simulink library "milstd_library"  (Simulink 6.0)
settings: Solver=ode45  SolverMode=SingleTasking  StartTime=0.0  StopTime=10.0  RelTol=1e-3
undefined symbols (not defined in the file or in its folder): milstd
libraries: simulink x13, commutil2 x11, dspsigattribs x6, dspbuff3 x5, commcnvcod2 x4, commseqgen2 x3, milstd_library x3, dspsigops x3, dspsrcs4 x3, dspmtrx3 x2, commdigbbndpm2 x2, commblkintrlv2 x2
settings Model: Creator=arodrigu  LastModifiedBy=arodrigu
settings DataIOCC: SignalLoggingName=logsOut
settings OptimizationCC: BooleanDataType=off
settings DebuggingCC: CheckExecutionContextPreStartOutputMsg=on  CheckExecutionContextRuntimeOutputMsg=on  SolverPrmCheckMsg=none
settings HardwareCC: TargetUnknown=on
settings ModelReferenceCC: UpdateModelReferenceTargets=IfOutOfDate
settings SFSimCC: SFSimApplyToAllLibs=on  SFSimBuildMode=Incremental

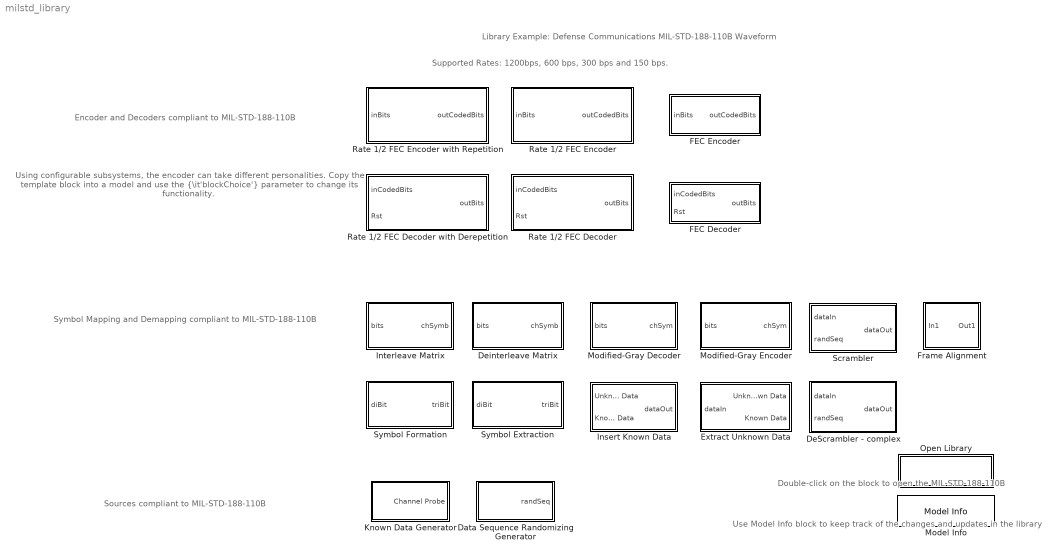
== system milstd_library ==
  note: Library Example: Defense Communications MIL-STD-188-110B Waveform
  note: Encoder and Decoders
      | compliant to
      | MIL-STD-188-110B
  note: Symbol Mapping and Demapping
      | compliant to
      | MIL-STD-188-110B
  note: Sources
      | compliant to
      | MIL-STD-188-110B
  note: Using configurable subsystems,
      | the encoder can take different
      | personalities. Copy the template block
      | into a model and use the {\it'blockChoice'}
      | parameter to change its functionality.
  note: Supported Rates: 1200bps, 600 bps, 300 bps and 150 bps.
  note: Use Model Info block to keep track of
      | the changes and updates in the library
  note: Double-click on the block
      | to open the MIL-STD-188-110B
  Data Sequence Randomizing Generator : Subsystem  PropExecContextAcrossSSBoundary=on
  DeScrambler - complex : Subsystem  PropExecContextAcrossSSBoundary=on
      mask Display:
      | disp('Descrambler\n')
      | port_label('input',1,'');
      | port_label('input',2,'rndSeq');
  Deinterleave Matrix : Subsystem  PropExecContextAcrossSSBoundary=on
      mask Display: disp('Deinterleave\nMatrix')
  Extract Unknown Data : Subsystem  PropExecContextAcrossSSBoundary=on
      mask Display: disp('Extract\nUnknown Data')
  FEC Decoder : Subsystem  BlockChoice=Rate 1/2 FEC Decoder  PropExecContextAcrossSSBoundary=on
      settings: TemplateBlock=self  MemberBlocks=Rate 1/2 FEC Decoder,Rate 1/2 FEC Decoder with Derepetition
  FEC Encoder : Subsystem  BlockChoice=Rate 1/2 FEC Encoder  PropExecContextAcrossSSBoundary=on
      settings: TemplateBlock=self  MemberBlocks=Rate 1/2 FEC Encoder,Rate 1/2 FEC Encoder with Repetition
  Frame Alignment : Subsystem  PropExecContextAcrossSSBoundary=on
      mask Display: disp('Frame\nAlignment')
  Insert Known Data : Subsystem  PropExecContextAcrossSSBoundary=on
      mask Display: disp('Insert\nKnown Data')
  Interleave Matrix : Subsystem  PropExecContextAcrossSSBoundary=on
      mask Display: disp('Interleave\nMatrix')
  Known Data Generator : Subsystem  PropExecContextAcrossSSBoundary=on
  Model Info : simulink/Model-Wide Utilities/Model Info  InitialBlockCM=None  BlockCM=None  Frame=on  DisplayStringWithTags=|  HorizontalTextAlignment=Center  LeftAlignmentValue=0.5  SourceBlockDiagram=milstd_library  TagMaxNumber=20
      | Model Info
      | Model version: %<ModelVersion>
  Modified-Gray Decoder : Subsystem  PropExecContextAcrossSSBoundary=on
      mask Display: disp('Bits to\nChannel\nSymbols')
  Modified-Gray Encoder : Subsystem  PropExecContextAcrossSSBoundary=on
      mask Type: Modified-Gray Encoder
      mask Display: disp('Channel\nSymbols\nto Bits')
  Open Library : Subsystem  PropExecContextAcrossSSBoundary=on
      settings: OpenFcn=open('milstd_188110bmodel.mdl');
      mask Display: disp('MIL-STD-188-110B\nModel')
  Rate 1/2 FEC Decoder : Subsystem  PropExecContextAcrossSSBoundary=on
      mask Display: disp('Rate 1/2\nFEC Decoding:\nViterbi Decoder');
  Rate 1/2 FEC Decoder with Derepetition : Subsystem  PropExecContextAcrossSSBoundary=on
      mask Display: disp('Rate 1/2\nFEC Decoding:\nViterbi Decoder\nwith Derepetition');
  Rate 1/2 FEC Encoder : Subsystem  PropExecContextAcrossSSBoundary=on
      mask Display: disp('Rate 1/2 FEC\nEncoder')
  Rate 1/2 FEC Encoder with Repetition : Subsystem  PropExecContextAcrossSSBoundary=on
      mask Display: disp('Rate 1/2 FEC\nEncoder\n with Repetition')
  Scrambler : Subsystem  PropExecContextAcrossSSBoundary=on
      mask Display:
      | disp('Scrambler')
      | port_label('input',1,'');
      | port_label('input',2,'rndSeq');
  Symbol Extraction : Subsystem  PropExecContextAcrossSSBoundary=on
      mask Display: disp('Symbol\nExtraction:\nUnknown Data')
  Symbol Formation : Subsystem  PropExecContextAcrossSSBoundary=on
      mask Display: disp('Symbol\nFormation:\nUnknown Data')

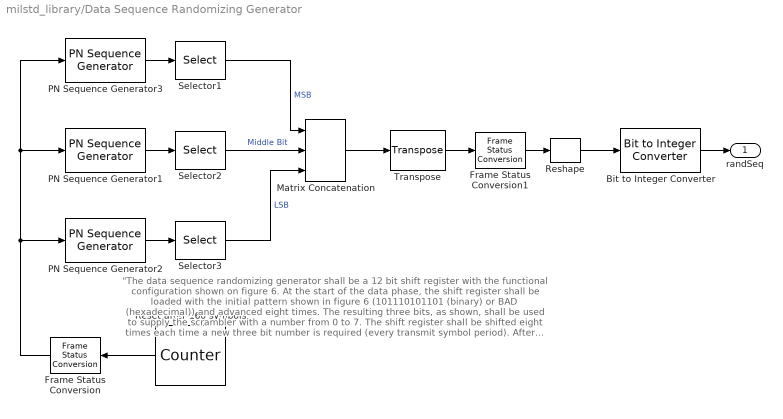
== system milstd_library/Data Sequence Randomizing Generator ==
  note: "The  data  sequence  randomizing  generator  shall  be  a  12  bit  shift  register  with  the  functional
      | configuration shown on figure 6. At the start of the data phase, the shift register shall be loaded
      | with the initial pattern shown in figure 6 (101110101101 (binary) or BAD (hexadecimal)) and
      | advanced eight times. The resulting three bits, as shown, shall be used to supply the scrambler
      | with a number from 0 to 7. The shift register shall be shifted eight times each time a new three
      | bit number is required  (every transmit symbol period). After 160 transmit symbols, the shift
      | register shall be reset to BAD (hexadecimal) prior to the eight shifts. "
      |
      | Source: MIL-STD-188-110B: Interoperability and Performance Standards for Data Modems,
      | U.S. Department of Defense, 2000.
  Bit to Integer Converter : commutil2/Bit to Integer Converter  nbits=3
  Frame Status Conversion : dspsigattribs/Frame Status Conversion  Orientation=left  growRefPort=off  outframe=Frame-based
  Frame Status Conversion1 : dspsigattribs/Frame Status Conversion  growRefPort=off  outframe=Frame-based
  Matrix Concatenation : simulink/Math Operations/Matrix Concatenation  numInports=3  catMethod=Horizontal
  PN Sequence Generator1 : commseqgen2/PN Sequence Generator  poly=[12 6 4 1 0]  ini_sta=[zeros(1,11) 1]  shift=3664  Ts=1/2400/8  frameBased=on  sampPerFrame=40*8  reset=on
  PN Sequence Generator2 : commseqgen2/PN Sequence Generator  poly=[12 6 4 1 0]  ini_sta=[zeros(1,11) 1]  shift=1506  Ts=1/2400/8  frameBased=on  sampPerFrame=40*8  reset=on
  PN Sequence Generator3 : commseqgen2/PN Sequence Generator  poly=[12 6 4 1 0]  ini_sta=[zeros(1,11) 1]  shift=3663  Ts=1/2400/8  frameBased=on  sampPerFrame=40*8  reset=on
  Reset after 160 symbols : dspswit3/Counter  Orientation=left  Direction=Down  CountEvent=Free running  CounterSize=User defined  MaxCount=160/40+1  InitialCount=160/40+1  Output=Hit  HitValue=1  ResetInput=off  SamplesPerFrame=1  Ts=40/2400  CntDtype=double  HitDtype=Logical
  Reshape : simulink/Math Operations/Reshape  OutputDimensionality=Column vector  OutputDimensions=[1,1]
  Selector1 : Selector  Elements=[8:8:40*8]  InputPortWidth=40*8
  Selector2 : Selector  Elements=[8:8:40*8]  InputPortWidth=40*8
  Selector3 : Selector  Elements=[8:8:40*8]  InputPortWidth=40*8
  Transpose : dspmtrx3/Transpose  Hermitian=off  overflowFlag=on
  randSeq : Outport
  wires:
  PN Sequence Generator2/1 -> Selector3/1
  PN Sequence Generator1/1 -> Selector2/1
  PN Sequence Generator3/1 -> Selector1/1
  Selector1/1 -> Matrix Concatenation/1  "MSB"
  Selector2/1 -> Matrix Concatenation/2  "Middle Bit"
  Selector3/1 -> Matrix Concatenation/3  "LSB"
  Bit to Integer Converter/1 -> randSeq/1
  Reset after 160 symbols/1 -> Frame Status Conversion/1
  Frame Status Conversion/1 -> PN Sequence Generator3/1, PN Sequence Generator1/1, PN Sequence Generator2/1
  Matrix Concatenation/1 -> Transpose/1
  Transpose/1 -> Frame Status Conversion1/1
  Reshape/1 -> Bit to Integer Converter/1
  Frame Status Conversion1/1 -> Reshape/1

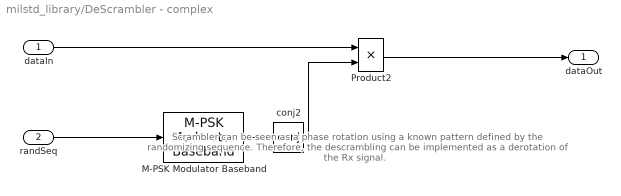
== system milstd_library/DeScrambler - complex ==
  note: Scrambler can be seen as a phase rotation using a known
      | pattern defined by the randomizing sequence. Therefore,
      | the descrambling can be implemented as a derotation of the
      | Rx signal.
  dataIn : Inport  LatchInput=off
  randSeq : Inport  Port=2  LatchInput=off
  M-PSK Modulator Baseband : commdigbbndpm2/M-PSK Modulator Baseband  M=8  InType=Integer  Enc=Binary  Ph=0  numSamp=1
  Product2 : Product  SaturateOnIntegerOverflow=on  InputSameDT=on
  conj2 : Math  Operator=conj  SaturateOnIntegerOverflow=on
  dataOut : Outport
  wires:
  Product2/1 -> dataOut/1
  conj2/1 -> Product2/2
  M-PSK Modulator Baseband/1 -> conj2/1
  randSeq/1 -> M-PSK Modulator Baseband/1
  dataIn/1 -> Product2/1

== system milstd_library/Deinterleave Matrix ==
  bits : Inport  LatchInput=off
  Buffer : dspbuff3/Buffer  N=milstd.rate*milstd.repFactor*2*0.2  V=0  ic=0
  General Block Deinterleaver : commblkintrlv2/General Block Deinterleaver  elements=milstd.interTable %Column vector
  chSymb : Outport
  wires:
  bits/1 -> General Block Deinterleaver/1
  General Block Deinterleaver/1 -> Buffer/1
  Buffer/1 -> chSymb/1

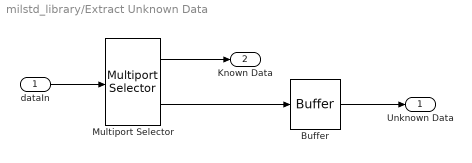
== system milstd_library/Extract Unknown Data ==
  dataIn : Inport  LatchInput=off
  Buffer : dspbuff3/Buffer  N=milstd.rate*2*milstd.interl*milstd.repFactor*3/milstd.bitsToSym  V=0  ic=0
  Multiport Selector : dspindex/Multiport Selector  rowsOrCols=Rows  idxCellArray={ [1:60],[61:120]}  idxErrMode=Clip Index
  Unknown Data : Outport
  Known Data : Outport  Port=2
  wires:
  dataIn/1 -> Multiport Selector/1
  Multiport Selector/1 -> Known Data/1
  Multiport Selector/2 -> Buffer/1
  Buffer/1 -> Unknown Data/1

== system milstd_library/FEC Decoder ==
  inCodedBits : Inport  LatchInput=off
  Rst : Inport  Port=2  LatchInput=off
  Rate 1/2 FEC Decoder : milstd_library/Rate 1//2 FEC Decoder
  outBits : Outport
  wires:
  inCodedBits/1 -> Rate 1/2 FEC Decoder/1
  Rst/1 -> Rate 1/2 FEC Decoder/2
  Rate 1/2 FEC Decoder/1 -> outBits/1

== system milstd_library/FEC Encoder ==
  inBits : Inport  LatchInput=off
  Rate 1/2 FEC Encoder : milstd_library/Rate 1//2 FEC Encoder
  outCodedBits : Outport
  wires:
  inBits/1 -> Rate 1/2 FEC Encoder/1
  Rate 1/2 FEC Encoder/1 -> outCodedBits/1

== system milstd_library/Frame Alignment ==
  note: This block collects a block
      | of data equal to size of the interleaver
      | matrix depending on the data rate and
      | interleaver length
  note: This extra delay is intended to
      | align the signal to the beginning of
      | the interleaver frame
  In1 : Inport  LatchInput=off
  Buffer : dspbuff3/Buffer  N=1200*milstd.interl  V=0  ic=0
  Delay : dspsigops/Delay  dly_unit=Samples  delay=1200*milstd.interl-20  ic_detail=off  dif_ic_for_ch=off  dif_ic_for_dly=off  ic=0  reset_popup=None
  Out1 : Outport
  wires:
  Delay/1 -> Buffer/1
  Buffer/1 -> Out1/1
  In1/1 -> Delay/1

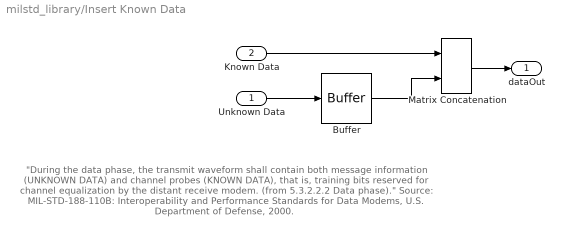
== system milstd_library/Insert Known Data ==
  note: "During  the  data  phase,  the  transmit  waveform  shall  contain  both  message  information
      | (UNKNOWN DATA) and channel probes (KNOWN DATA), that is, training bits reserved for
      | channel equalization by the distant receive modem. (from 5.3.2.2.2 Data phase)."
      |
      | Source: MIL-STD-188-110B: Interoperability and Performance Standards for Data Modems,
      | U.S. Department of Defense, 2000.
  Unknown Data : Inport  LatchInput=off
  Known Data : Inport  Port=2  LatchInput=off
  Buffer : dspbuff3/Buffer  N=20*3  V=0  ic=0
  Matrix Concatenation : simulink/Math Operations/Matrix Concatenation  numInports=2  catMethod=Vertical
  dataOut : Outport
  wires:
  Buffer/1 -> Matrix Concatenation/2
  Known Data/1 -> Matrix Concatenation/1
  Matrix Concatenation/1 -> dataOut/1
  Unknown Data/1 -> Buffer/1

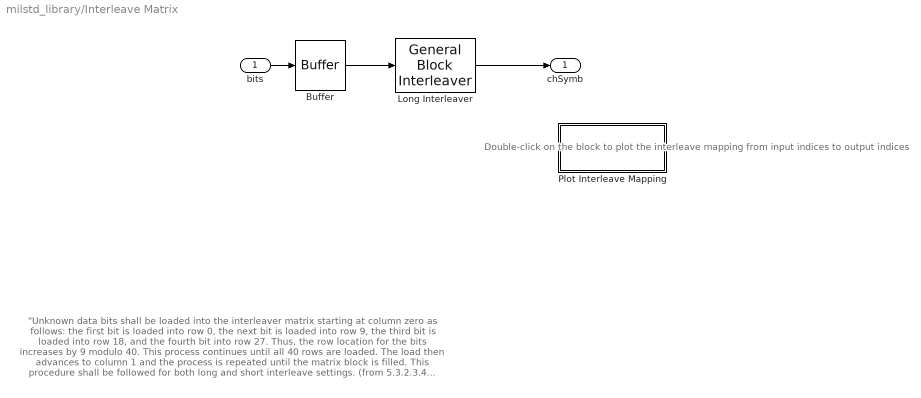
== system milstd_library/Interleave Matrix ==
  note: "Unknown data bits shall be loaded into the interleaver matrix starting at column zero as follows:
      | the first bit is loaded into row 0, the next bit is loaded into row 9, the third bit is loaded into row 18, and the fourth
      | bit into row 27. Thus, the row location for the bits increases by 9 modulo 40. This process continues until all 40 rows
      | are loaded. The load then advances to column 1 and the process is repeated until the matrix block is filled. This procedure
      | shall be followed for both long and short interleave settings. (from 5.3.2.3.4 Interleave load).
      |
      | To maintain the interleave delay at a constant value, the block size shall be scaled by bit rate. TABLES X lists the interleaver
      | matrix dimensions (rows and columns) that shall be allocated for each requir d bit rate and interleave delay.
      |
      | The fetching sequence for all rates shall start with the first bit being taken from row zero, column zero. The location of
      | each successive fetched bit shall be determined by incrementing the row by one and decrementing the column
      | number by 17 (modulo number of columns in the interleaver matrix).  (from 5.3.2.3.5 Interleave fetch)."
      |
      | Source: MIL-STD-188-110B: Interoperability and Performance Standards for Data Modems, U.S. Department of Defense, 2000.
  note: Double-click on the block to
      | plot the interleave mapping from
      | input indices to output indices
  bits : Inport  LatchInput=off
  Buffer : dspbuff3/Buffer  N=milstd.rate*milstd.interl*milstd.repFactor*2 % x2 because of coding rate  V=0  ic=0
  Long Interleaver : commblkintrlv2/General Block Interleaver  elements=milstd.interTable %Column vector
  Plot Interleave Mapping : Subsystem  PropExecContextAcrossSSBoundary=on
      settings: OpenFcn=|
      | figure;
      | numRow = 40;
      | numCol = length(milstd.interTable)/numRow;
      | plot([0:numRow*numCol-1],milstd.interTable,'b.');
      | axis([0 numRow*numCol-1 0 numRow*numCol-1]);
      | title('Interleaver Mapping');
      | xlabel('Input index');
      | ylabel('Output index');
      mask Display: disp('Interleave\nMapping')
  chSymb : Outport
  wires:
  Long Interleaver/1 -> chSymb/1
  Buffer/1 -> Long Interleaver/1
  bits/1 -> Buffer/1

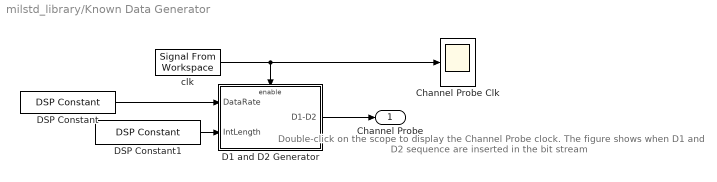
== system milstd_library/Known Data Generator ==
  note: Double-click on the scope to display
      | the Channel Probe clock. The figure shows
      | when D1 and D2 sequence are inserted in
      | the bit stream
  Channel Probe Clk : Scope
      settings: TimeRange=19.2  DataFormat=Structure
  D1 and D2 Generator : Subsystem  PropExecContextAcrossSSBoundary=on
      mask init:
      | % Loads lookup table for D1 and D2 bits in preamble sequence
      | % according to MIL-STD-188-110B TABLE XV
      | % D1 Lookup table:
      | D1Table = ones(7,2);
      | D1Table(:,1) = [ 7 6 6 6 6 7 7]';
      | D1Table(:,2) = [ 0 4 4 4 4 5 5]';
      | 
      | % D1 Lookup table:
      | D2Table = ones(7,2);
      | D2Table(:,1) = [6 4 5 6 7 4 5]';
      | D2Table(:,2) = [0 4 5 6 7 4 5]';
  DSP Constant : dspsrcs4/DSP Constant  Value=milstd.idxRate  SampleMode=Discrete  discreteOutput=Frame-based  continuousOutput=Sample-based  sampTime=1  framePeriod=20/1200  dataType=Inherit from 'Constant value'  wordLen=16  udDataType=sfix(16)  fracBitsMode=Best precision  numFracBits=15  InterpretAs1D=-inf  Ts=-inf  FramebasedOutput=-inf
  DSP Constant1 : dspsrcs4/DSP Constant  Value=milstd.idxInterl  SampleMode=Discrete  discreteOutput=Frame-based  continuousOutput=Sample-based  sampTime=1  framePeriod=20/1200  dataType=Inherit from 'Constant value'  wordLen=16  udDataType=sfix(16)  fracBitsMode=Best precision  numFracBits=15  InterpretAs1D=-inf  Ts=-inf  FramebasedOutput=-inf
  clk : dspsrcs4/Signal From Workspace  X="[1 1 zeros(1,1200*milstd.rate/20-2)]  %Channel rate is equal to 1200"  Ts=20/1200  nsamps=1  OutputAfterFinalValue=Cyclic repetition
  Channel Probe : Outport
  wires:
  clk/1 -> D1 and D2 Generator/Enable, Channel Probe Clk/1
  DSP Constant/1 -> D1 and D2 Generator/1(DataRate)
  DSP Constant1/1 -> D1 and D2 Generator/2(IntLength)
  D1 and D2 Generator/1(D1-D2) -> Channel Probe/1

== system milstd_library/Modified-Gray Decoder ==
  note: The bits obtained from the interleaver matrix shall be
      | grouped together as one, two, or three bit
      | entities that will be referred to as channel symbols.
  note: "Modified-Gray decoding of the 2400 bps, 4800 bps (tribit), and 75 bps (fixed frequency) 1200
      | bps (dibit) channel symbols shall be in accordance with tables XII and XIII respectively. "
      |
      | Source: MIL-STD-188-110B: Interoperability and Performance Standards for Data Modems, U.S. Department of Defense, 2000.
  bits : Inport  LatchInput=off
  Bits to Channel symbols : commutil2/Bit to Integer Converter  nbits=milstd.bitsToSym
  Data Mapper : commutil2/Data Mapper  MapMode=Binary to Gray  M=2^milstd.bitsToSym  MapVec=[0 1 3 2]
  Integer to Bit Converter : commutil2/Integer to Bit Converter  nbits=milstd.bitsToSym
  chSym : Outport
  wires:
  Data Mapper/1 -> Integer to Bit Converter/1
  bits/1 -> Bits to Channel symbols/1
  Integer to Bit Converter/1 -> chSym/1
  Bits to Channel symbols/1 -> Data Mapper/1

== system milstd_library/Modified-Gray Encoder ==
  bits : Inport  LatchInput=off
  Bits to Channel symbols : commutil2/Bit to Integer Converter  nbits=milstd.bitsToSym
  Data Mapper : commutil2/Data Mapper  MapMode=Gray to Binary  M=2^milstd.bitsToSym  MapVec=[0 1 3 2]
  Integer to Bit Converter : commutil2/Integer to Bit Converter  nbits=milstd.bitsToSym
  chSym : Outport
  wires:
  Bits to Channel symbols/1 -> Data Mapper/1
  Integer to Bit Converter/1 -> chSym/1
  bits/1 -> Bits to Channel symbols/1
  Data Mapper/1 -> Integer to Bit Converter/1

== system milstd_library/Open Library ==
  note: This subsystem is intentionally left empty

== system milstd_library/Rate 1/2 FEC Decoder ==
  inCodedBits : Inport  Orientation=left  LatchInput=off
  Rst : Inport  Orientation=left  Port=2  LatchInput=off
  Rate 1/2 Viterbi Decoder : commcnvcod2/Viterbi Decoder  Orientation=left  trellis=poly2trellis(7, [133 171])  dectype=Hard Decision  nsdecb=4  tbdepth=34  opmode=Continuous  reset=on
  outBits : Outport  Orientation=left
  wires:
  inCodedBits/1 -> Rate 1/2 Viterbi Decoder/1
  Rst/1 -> Rate 1/2 Viterbi Decoder/2
  Rate 1/2 Viterbi Decoder/1 -> outBits/1

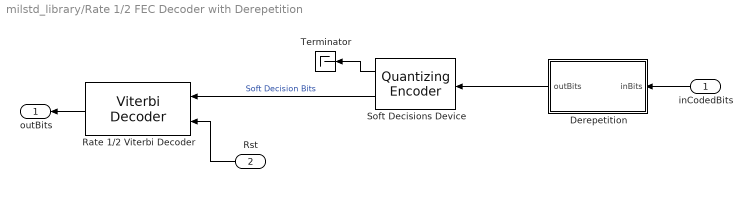
== system milstd_library/Rate 1/2 FEC Decoder with Derepetition ==
  inCodedBits : Inport  Orientation=left  LatchInput=off
  Rst : Inport  Orientation=left  Port=2  LatchInput=off
  Derepetition : Subsystem  Orientation=left  PropExecContextAcrossSSBoundary=on
      mask Display: disp('Derepetition')
  Rate 1/2 Viterbi Decoder : commcnvcod2/Viterbi Decoder  Orientation=left  trellis=poly2trellis(7, [133 171])  dectype=Soft Decision  nsdecb=2  tbdepth=34  opmode=Continuous  reset=on
  Soft Decisions Device : commsrccod2/Quantizing Encoder  Orientation=left  partition=[0.1 0.5 0.9]*milstd.repFactor  codebook=[0 1 2 3]
  Terminator : Terminator
  outBits : Outport  Orientation=left
  wires:
  Rate 1/2 Viterbi Decoder/1 -> outBits/1
  Rst/1 -> Rate 1/2 Viterbi Decoder/2
  inCodedBits/1 -> Derepetition/1(inBits)
  Derepetition/1(outBits) -> Soft Decisions Device/1
  Soft Decisions Device/1 -> Terminator/1
  Soft Decisions Device/2 -> Rate 1/2 Viterbi Decoder/1  "Soft Decision Bits"

== system milstd_library/Rate 1/2 FEC Encoder ==
  note: "The FEC encoder shall be used for data rates up to and including 2400 bps. [...] For
      | frequency-hopping operation, the FEC encoder function shall be accomplished by a constraint
      | length 7 convolutional coder with repeat coding used at the 75, 150, and 300 bps rates.
      |
      | The two summing nodes on the figure represent modulo 2 addition. For each bit input to the encoder, two
      | bits shall be taken as output from the encoder, the upper output bit Tl(x) being taken first. [...]
      | At all other rates, the convolutional coder shall be rate 1/2.
      |
      | Coded bit streams of 3600, 2400, and 1200 bps shall be generated for the input data rates of 2400, 1200, and 600 bps, respectively.
      | For the 300, 150, and 75 bps input data rates, a 1200 bps coded bit  stream shall be generated by repeating the pairs of output bits the
      | appropriate number  of  times.
      |
      | The  bits  shall  be  repeated  in  pairs  rather  than  repetitions  for  the first, Tl(x), followed  by repetitions of the second T2(x).
      | (from 5.3.2.3.3 FEC encoder.)."
      |
      | Source: MIL-STD-188-110B: Interoperability and Performance Standards for Data Modems, U.S. Department of Defense, 2000.
  note: Double-click on the block to
      | compare the convolutional encoder
      | realization in the Communications
      | Blockset with the block diagram
      | representation specified by the
      | standard
  inBits : Inport  LatchInput=off
  Compare FEC Encoder Implementation : Subsystem  PropExecContextAcrossSSBoundary=on
      settings: OpenFcn=|
      | if(which('milstd_TestEncoderFigure4'))
      | open('milstd_TestEncoderFigure4');
      | else
      | errordlg('File milstd_TestEncoderFigure4.mdl not found.');
      | end
      mask Display: disp('Compare\nFEC Encoder')
  Rate 1/2 FEC Encoder : commcnvcod2/Convolutional Encoder  trellis=poly2trellis(7, [133 171])  reset=None
  outCodedBits : Outport
  wires:
  inBits/1 -> Rate 1/2 FEC Encoder/1
  Rate 1/2 FEC Encoder/1 -> outCodedBits/1

== system milstd_library/Rate 1/2 FEC Encoder with Repetition ==
  note: "The FEC encoder shall be used for data rates up to and including 2400 bps. [...] For
      | frequency-hopping operation, the FEC encoder function shall be accomplished by a constraint
      | length 7 convolutional coder with repeat coding used at the 75, 150, and 300 bps rates.
      |
      | The two summing nodes on the figure represent modulo 2 addition. For each bit input to the encoder, two
      | bits shall be taken as output from the encoder, the upper output bit Tl(x) being taken first. [...]
      | At all other rates, the convolutional coder shall be rate 1/2.
      |
      | Coded bit streams of 3600, 2400, and 1200 bps shall be generated for the input data rates of 2400, 1200, and 600 bps, respectively.
      | For the 300, 150, and 75 bps input data rates, a 1200 bps coded bit  stream shall be generated by repeating the pairs of output bits the
      | appropriate number  of  times.
      |
      | The  bits  shall  be  repeated  in  pairs  rather  than  repetitions  for  the first, Tl(x), followed  by repetitions of the second T2(x).
      | (from 5.3.2.3.3 FEC encoder.)."
      |
      | Source: MIL-STD-188-110B: Interoperability and Performance Standards for Data Modems, U.S. Department of Defense, 2000.
  note: Double-click on the block to
      | compare the convolutional encoder
      | realization in the Communications
      | Blockset with the block diagram
      | representation specified by the
      | standard
  inBits : Inport  LatchInput=off
  Compare FEC Encoder Implementation : milstd_library/Rate 1//2 FEC Encoder/Compare FEC Encoder Implementation
  Rate 1/2 FEC Encoder : commcnvcod2/Convolutional Encoder  trellis=poly2trellis(7, [133 171])  reset=None
  Repeat xTimes : Subsystem  PropExecContextAcrossSSBoundary=on
      mask Display: disp('Repeat pairs\n xTimes')
  outCodedBits : Outport
  wires:
  Rate 1/2 FEC Encoder/1 -> Repeat xTimes/1(In1)
  inBits/1 -> Rate 1/2 FEC Encoder/1
  Repeat xTimes/1(Out1) -> outCodedBits/1

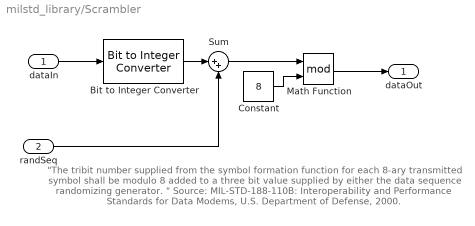
== system milstd_library/Scrambler ==
  note: "The tribit number supplied from the symbol formation function for each 8-ary transmitted
      | symbol shall be modulo 8 added to a three bit value supplied by either the data sequence
      | randomizing generator. "
      |
      | Source: MIL-STD-188-110B: Interoperability and Performance Standards for Data Modems, U.S.
      | Department of Defense, 2000.
  dataIn : Inport  LatchInput=off
  randSeq : Inport  Port=2  LatchInput=off
  Bit to Integer Converter : commutil2/Bit to Integer Converter  nbits=3 %Tribit input
  Constant : Constant  Value=8
  Math Function : Math  Operator=mod  SaturateOnIntegerOverflow=on
  Sum : Sum  Inputs=|++  SaturateOnIntegerOverflow=on
  dataOut : Outport
  wires:
  dataIn/1 -> Bit to Integer Converter/1
  Bit to Integer Converter/1 -> Sum/1
  randSeq/1 -> Sum/2
  Sum/1 -> Math Function/1
  Math Function/1 -> dataOut/1
  Constant/1 -> Math Function/2

== system milstd_library/Symbol Extraction ==
  note: "The function of the symbol extraction is to convert the tribit that results from the modulation into
      | one, two, or three bit channel symbols depending on the data rate."
      |
      | Source: MIL-STD-188-110B: Interoperability and Performance Standards for Data Modems, U.S. Department of Defense, 2000.
  diBit : Inport  LatchInput=off
  M-PSK Demodulator Baseband : commdigbbndpm2/M-PSK Demodulator Baseband  M=2^(milstd.bitsToSym)  OutType=Bit  Dec=Binary  Ph=0  numSamp=1
  triBit : Outport
  wires:
  M-PSK Demodulator Baseband/1 -> triBit/1
  diBit/1 -> M-PSK Demodulator Baseband/1

== system milstd_library/Symbol Formation ==
  note: "The function of symbol formation is one of mapping the one, two, or three bit channel symbols
      | from  the  MGD  into  tribit  numbers  compatible with transmission using an 8-ary modulation scheme.
      | (from 5.3.2.3.7 Symbol formation).
      |
      | When one bit channel symbols are used (600-150 bps), the symbol formation output shall be
      | tribit numbers 0 and 4 At the 1200-bps rate, the dibit channel symbol formation shall use tribit numbers 0, 2, 4, and 6."
      |
      | Source: MIL-STD-188-110B: Interoperability and Performance Standards for Data Modems, U.S. Department of Defense, 2000.
  diBit : Inport  LatchInput=off
  Bit to Integer Converter : commutil2/Bit to Integer Converter  nbits=milstd.bitsToSym
  Integer to Bit Converter : commutil2/Integer to Bit Converter  nbits=3 %Tribit output
  Shift Left : Gain  Gain=2^(3-milstd.bitsToSym)  SaturateOnIntegerOverflow=on
  triBit : Outport
  wires:
  Shift Left/1 -> Integer to Bit Converter/1
  Bit to Integer Converter/1 -> Shift Left/1
  diBit/1 -> Bit to Integer Converter/1
  Integer to Bit Converter/1 -> triBit/1

== system milstd_library/Interleave Matrix/Plot Interleave Mapping ==

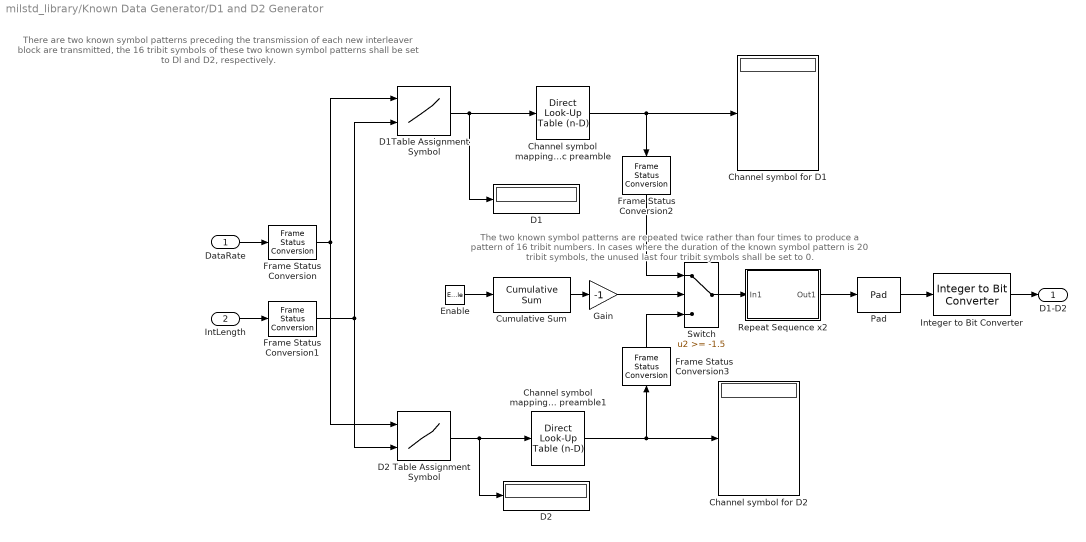
== system milstd_library/Known Data Generator/D1 and D2 Generator ==
  note: The two known symbol patterns are repeated twice rather than four times
      | to produce a pattern of 16 tribit numbers.  In cases where the duration of the
      | known symbol pattern is 20 tribit symbols, the unused last four tribit symbols shall be set to 0.
  note: There are two known symbol patterns preceding the transmission of each new
      | interleaver block are transmitted, the 16 tribit symbols of these two known symbol patterns shall
      | be set to Dl and D2, respectively.
  DataRate : Inport  LatchInput=off
  IntLength : Inport  Port=2  LatchInput=off
  Enable : EnablePort  StatesWhenEnabling=reset  ShowOutputPort=on
  Channel symbol for D1 : Display
  Channel symbol for D2 : Display
  Channel symbol mapping for sync preamble : simulink/Look-Up Tables/Direct Look-Up Table (n-D)  maskTabDims=2  explicitNumDims=1  outDims=Column  tabIsInput=off  mxTable=milstd.chSymMapping  clipFlag=Error
  Channel symbol mapping for sync preamble1 : simulink/Look-Up Tables/Direct Look-Up Table (n-D)  maskTabDims=2  explicitNumDims=1  outDims=Column  tabIsInput=off  mxTable=milstd.chSymMapping  clipFlag=Warning
  Cumulative Sum : dspmathops/Cumulative Sum  dim=Channels (running sum)  reset_popup=None
  D1 : Display
  D1Table Assignment Symbol : Lookup2D  DialogController=Simulink.DDGSource  RowIndex=[1:7]  ColumnIndex=[1:2]  OutputValues=milstd.D1Table  SaturateOnIntegerOverflow=on
  D2 : Display
  D2 Table Assignment Symbol : Lookup2D  DialogController=Simulink.DDGSource  RowIndex=[1:7]  ColumnIndex=[1:2]  OutputValues=milstd.D2Table  SaturateOnIntegerOverflow=on
  Frame Status Conversion : dspsigattribs/Frame Status Conversion  growRefPort=off  outframe=Sample-based
  Frame Status Conversion1 : dspsigattribs/Frame Status Conversion  growRefPort=off  outframe=Sample-based
  Frame Status Conversion2 : dspsigattribs/Frame Status Conversion  Orientation=down  growRefPort=off  outframe=Frame-based
  Frame Status Conversion3 : dspsigattribs/Frame Status Conversion  Orientation=up  growRefPort=off  outframe=Frame-based
  Gain : Gain  Gain=-1  SaturateOnIntegerOverflow=on
  Integer to Bit Converter : commutil2/Integer to Bit Converter  nbits=3
  Pad : dspsigops/Pad  padVal=0  padSigAt=End  padAlong=Columns  padNumOutRowsSpecMethod=User-specified  numOutRows=20  padNumOutColsSpecMethod=User-specified  numOutCols=1  trunc_flag=None
  Repeat Sequence x2 : Subsystem  PropExecContextAcrossSSBoundary=on
      mask Display: disp('Repeat\nSequence x2')
  Switch : Switch  Threshold=-1.5  SaturateOnIntegerOverflow=on
  D1-D2 : Outport  OutputWhenDisabled=reset  InitialOutput=0
  wires:
  DataRate/1 -> Frame Status Conversion/1
  IntLength/1 -> Frame Status Conversion1/1
  D1Table Assignment Symbol/1 -> Channel symbol mapping for sync preamble/1, D1/1
  D2 Table Assignment Symbol/1 -> Channel symbol mapping for sync preamble1/1, D2/1
  Channel symbol mapping for sync preamble/1 -> Channel symbol for D1/1, Frame Status Conversion2/1
  Channel symbol mapping for sync preamble1/1 -> Channel symbol for D2/1, Frame Status Conversion3/1
  Frame Status Conversion/1 -> D2 Table Assignment Symbol/1, D1Table Assignment Symbol/1
  Frame Status Conversion1/1 -> D2 Table Assignment Symbol/2, D1Table Assignment Symbol/2
  Repeat Sequence x2/1(Out1) -> Pad/1
  Pad/1 -> Integer to Bit Converter/1
  Switch/1 -> Repeat Sequence x2/1(In1)
  Frame Status Conversion3/1 -> Switch/3
  Frame Status Conversion2/1 -> Switch/1
  Enable/1 -> Cumulative Sum/1
  Cumulative Sum/1 -> Gain/1
  Integer to Bit Converter/1 -> D1-D2/1
  Gain/1 -> Switch/2

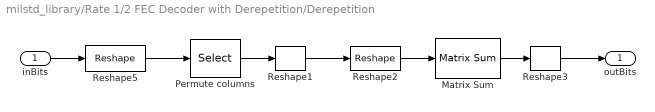
== system milstd_library/Rate 1/2 FEC Decoder with Derepetition/Derepetition ==
  inBits : Inport  LatchInput=off
  Matrix Sum : dspmtrx3/Matrix Sum  Dim=Columns
  Permute columns : Selector  InputType=Matrix  Elements=[1 3]  Rows=[[1:2:2*milstd.repFactor] [2:2:2*milstd.repFactor]]  Columns=-1  InputPortWidth=3
  Reshape1 : simulink/Math Operations/Reshape  OutputDimensionality=Column vector  OutputDimensions=[2*milstd.repFactor,milstd.rate*0.2]
  Reshape2 : simulink/Math Operations/Reshape  OutputDimensionality=Customize  OutputDimensions=[milstd.repFactor,milstd.rate*0.2*2]
  Reshape3 : simulink/Math Operations/Reshape  OutputDimensionality=Column vector  OutputDimensions=[2*milstd.repFactor,milstd.rate*0.2]
  Reshape5 : simulink/Math Operations/Reshape  OutputDimensionality=Customize  OutputDimensions=[2*milstd.repFactor,milstd.rate*0.2]
  outBits : Outport
  wires:
  Reshape5/1 -> Permute columns/1
  Permute columns/1 -> Reshape1/1
  Reshape1/1 -> Reshape2/1
  Reshape2/1 -> Matrix Sum/1
  Matrix Sum/1 -> Reshape3/1
  inBits/1 -> Reshape5/1
  Reshape3/1 -> outBits/1

== system milstd_library/Rate 1/2 FEC Encoder/Compare FEC Encoder Implementation ==

== system milstd_library/Rate 1/2 FEC Encoder with Repetition/Repeat xTimes ==
  In1 : Inport  LatchInput=off
  Reshape5 : simulink/Math Operations/Reshape  OutputDimensionality=Customize  OutputDimensions=[2,milstd.rate*0.2]
  Reshape6 : simulink/Math Operations/Reshape  OutputDimensionality=Column vector  OutputDimensions=[1,1]
  Selector1 : Selector  InputType=Matrix  Elements=[1 3]  Rows=repmat([1 2],1,milstd.repFactor)  Columns=-1  InputPortWidth=3
  Out1 : Outport
  wires:
  Selector1/1 -> Reshape6/1
  Reshape5/1 -> Selector1/1
  In1/1 -> Reshape5/1
  Reshape6/1 -> Out1/1

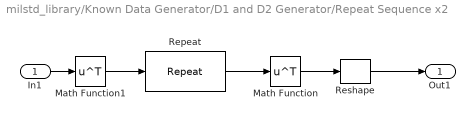
== system milstd_library/Known Data Generator/D1 and D2 Generator/Repeat Sequence x2 ==
  In1 : Inport  LatchInput=off
  Math Function : Math  Operator=transpose  SaturateOnIntegerOverflow=on
  Math Function1 : Math  Operator=transpose  SaturateOnIntegerOverflow=on
  Repeat : dspsigops/Repeat  N=2  ic=0  mode=Maintain input frame rate
  Reshape : simulink/Math Operations/Reshape  OutputDimensionality=Column vector  OutputDimensions=[1,1]
  Out1 : Outport
  wires:
  Repeat/1 -> Math Function/1
  Math Function/1 -> Reshape/1
  Math Function1/1 -> Repeat/1
  In1/1 -> Math Function1/1
  Reshape/1 -> Out1/1
